simulink model "oppg3_mekanikk_simulink"  (R2024a)
settings: Solver=VariableStepAuto  StartTime=0.0  StopTime=300  MaxStep=0.01  RelTol=1e-3
values from neighbouring files (symbols this model uses):
  d = 0.1    [oppg3_mekanikk.m]
  k = 1    [heron.m]    (also in oppg3_mekanikk.m)
  m = 1    [oppg3_mekanikk.m]
settings Model: Creator=filip  LastModifiedBy=filip

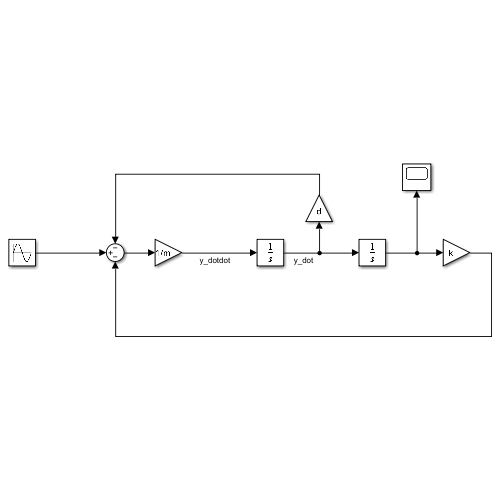
[thumbnail: Simulink's stored preview of the top-level diagram]
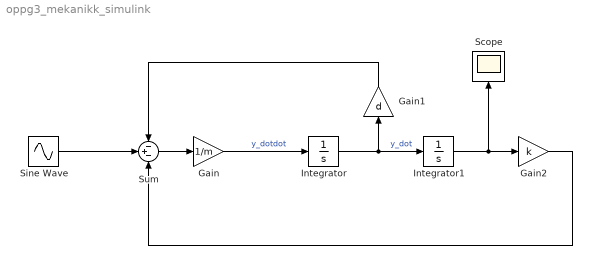
== system oppg3_mekanikk_simulink ==
  Gain : Gain  Gain=1/m
  Gain1 : Gain  Gain=d
  Gain2 : Gain  Gain=k
  Integrator : Integrator
  Integrator1 : Integrator  InitialCondition=1
  Scope : Scope
  Sine Wave : Sin  SampleTime=0
  Sum : Sum  Inputs=-+-
  wires:
  Sum/1 -> Gain/1
  Gain/1 -> Integrator/1  "y_dotdot"
  Integrator/1 -> Gain1/1, Integrator1/1  "y_dot"
  Integrator1/1 -> Scope/1, Gain2/1
  Gain2/1 -> Sum/3
  Gain1/1 -> Sum/1
  Sine Wave/1 -> Sum/2
